simulink model "comparison2"  (R2015b)
settings: Solver=VariableStepAuto  StartTime=0.0  StopTime=20  FixedStep=1e-3  MaxStep=1e-4  MinStep=1e-5  RelTol=1e-6
settings Model: Creator=dell  LastModifiedBy=dell

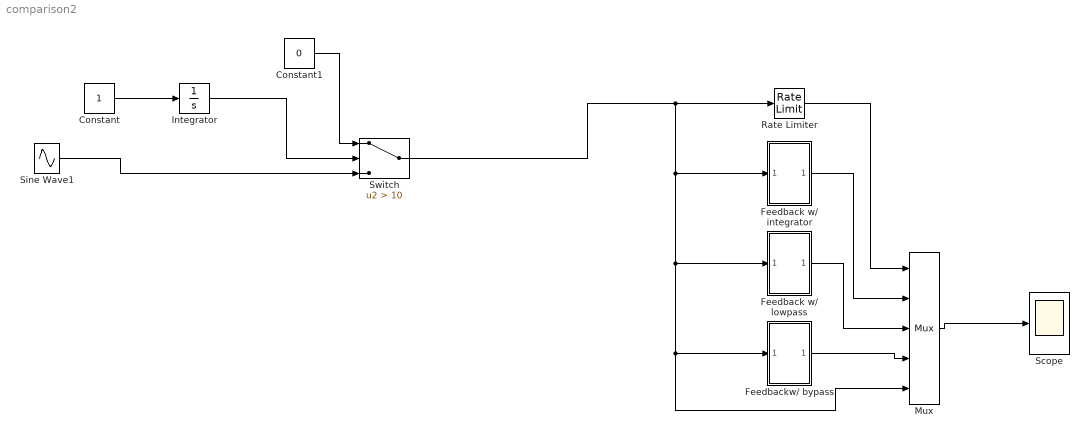
== system comparison2 ==
  Constant : Constant
  Constant1 : Constant  Value=0
  Feedback w/ integrator : Subsystem
  "Feedback w/ lowpass " : Subsystem
  Feedbackw/ bypass : Subsystem
  Integrator : Integrator
  Mux : Mux  Inputs=5
  Rate Limiter : RateLimiter  SampleTimeMode=inherited
  Scope : Scope
  Sine Wave1 : Sin  Amplitude=5  SampleTime=0
  Switch : Switch  Criteria=u2 > Threshold  Threshold=10
  wires:
  Mux/1 -> Scope/1
  Rate Limiter/1 -> Mux/1
  Feedback w/ integrator/1(Out1) -> Mux/2
  "Feedback w/ lowpass "/1(Out1) -> Mux/3
  Feedbackw/ bypass/1(Out1) -> Mux/4
  Constant/1 -> Integrator/1
  Integrator/1 -> Switch/2
  Sine Wave1/1 -> Switch/3
  Switch/1 -> Mux/5, Feedbackw/ bypass/1(In1), "Feedback w/ lowpass "/1(In1), Feedback w/ integrator/1(In1), Rate Limiter/1
  Constant1/1 -> Switch/1

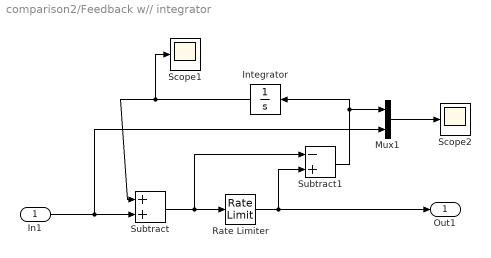
== system comparison2/Feedback w// integrator ==
  In1 : Inport
  Integrator : Integrator
  Mux1 : Mux  Inputs=2
  Rate Limiter : RateLimiter  SampleTimeMode=inherited
  Scope1 : Scope
  Scope2 : Scope
  Subtract : Sum
  Subtract1 : Sum  Inputs=-+
  Out1 : Outport
  wires:
  Rate Limiter/1 -> Out1/1, Subtract1/2
  Subtract1/1 -> Mux1/1, Integrator/1
  Integrator/1 -> Scope1/1, Subtract/1
  Subtract/1 -> Subtract1/1, Rate Limiter/1
  In1/1 -> Mux1/2, Subtract/2
  Mux1/1 -> Scope2/1

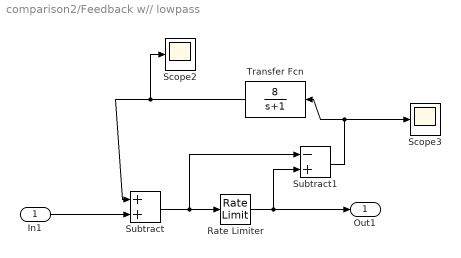
== system comparison2/Feedback w// lowpass  ==
  In1 : Inport
  Rate Limiter : RateLimiter  SampleTimeMode=inherited
  Scope2 : Scope
  Scope3 : Scope
  Subtract : Sum
  Subtract1 : Sum  Inputs=-+
  Transfer Fcn : TransferFcn  Numerator=[8]  Denominator=[1 1]
  Out1 : Outport
  wires:
  Subtract/1 -> Subtract1/1, Rate Limiter/1
  Rate Limiter/1 -> Out1/1, Subtract1/2
  Subtract1/1 -> Scope3/1, Transfer Fcn/1
  In1/1 -> Subtract/2
  Transfer Fcn/1 -> Scope2/1, Subtract/1

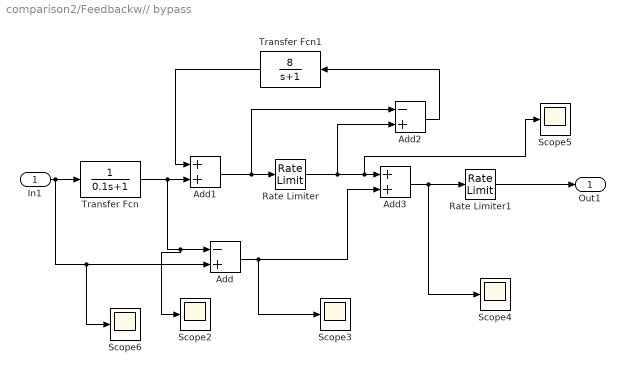
== system comparison2/Feedbackw// bypass ==
  In1 : Inport
  Add : Sum  Inputs=-+
  Add1 : Sum
  Add2 : Sum  Inputs=-+
  Add3 : Sum
  Rate Limiter : RateLimiter  SampleTimeMode=inherited
  Rate Limiter1 : RateLimiter  SampleTimeMode=inherited
  Scope{2..6} (5 alike) : Scope
  Transfer Fcn : TransferFcn  Denominator=[0.1 1]
  Transfer Fcn1 : TransferFcn  Numerator=[8]  Denominator=[1 1]
  Out1 : Outport
  wires:
  Rate Limiter1/1 -> Out1/1
  Add2/1 -> Transfer Fcn1/1
  Add/1 -> Scope3/1, Add3/2
  Add3/1 -> Scope4/1, Rate Limiter1/1
  Transfer Fcn/1 -> Scope2/1, Add/1, Add1/2
  Rate Limiter/1 -> Add2/2, Scope5/1, Add3/1
  In1/1 -> Scope6/1, Add/2, Transfer Fcn/1
  Add1/1 -> Add2/1, Rate Limiter/1
  Transfer Fcn1/1 -> Add1/1
